simulink model "CM13_2024a_MachE_for_UA_HIL"  (R2024a)
settings: Solver=ode1  StartTime=0.0  StopTime=Inf  FixedStep=0.001  RelTol=1e-3  EnableMultiTasking=on
PreLoadFcn:
  | % if ~length(which('cmcmd')), cmenv; end
PostLoadFcn:
  | if any(exist('dsrtsu_mdlpostloadfcn', 'file') ~= 0), dsrtsu_mdlpostloadfcn('Execute', bdroot); end
InitFcn:
  | , if any(exist('rtifpga_mdlclblib', 'file') ~= 0), rtifpga_mdlclblib('Init', bdroot); end,
  | , if any(exist('dsmpb_private', 'file') ~= 0), dsmpb_private('dsmpb_mdlclblib', 'Init', bdroot); end,
values from neighbouring files (symbols this model uses):
  CoastDown =     [Run_Simulink.mat]
  limitedMCT =     [Run_Simulink.mat]
  MCT =     [Run_Simulink.mat]
  pMCT =     [Run_Simulink.mat]
  RealSimPara =     [Run_Simulink.mat]
  Ref_speed = [13 13.007895099 13.015778396 13.023649891 13.031509584 13.039357475 13.047193564 13.055017851 13.062830336 13.070631019 13.0784199 13.086196979 ... (2669 elements, 2669x1)]    [Ref_speed_and_time.mat]
  Ref_time = [0 0.01 0.02 0.03 0.04 0.05 0.06 0.07 0.08 0.09 0.1 0.11 ... (2669 elements, 2669x1)]    [Ref_speed_and_time.mat]
  US06 =     [Run_Simulink.mat]
undefined symbols (not defined in the file or in its folder): AccelCmd, ActTqLF_Nm_, ActTqLR_Nm_, ActTqRF_Nm_, ActTqRR_Nm_, BattChargeLimitMaxPwr, BattChargeLimitSocBpts, BattChargeLimitTbl, BattChrgCapcty, BattDischargeLimitSocBpts, BattDischargeLimitTbl, BattDischargeMaxPwr, BattNumCellsParallel, BattNumCellsSeries, BattOpenVoltCapBpts, BattOpenVoltTbl, BattResistSocBpts, BattResistTbl, BattResistTempBpts, BrakeMaxPrs, BrakeMaxTrq, ChassisDistCg2FrontAxle, ChassisDistCg2RearAxle, ChassisVehMass, CltchCmd, DecelCmd, DiffRatio, DiscIntNeverNeededParam, EnvGravCnst, EnvPrs, EnvTemp, FuelSpecificGrav, GearCmd, h, InitStates, lgSw, MtrEffSpdBpts, MtrEffTbl, MtrEffTrqBpts, MtrPwrMax, MtrTrqMax, planned_speed, planned_time, ref_speed, ref_time, rticanmm_blockfcn, rticanmm_initfcn, SteeringCmd, SupvsryCtrlRegenBrkCutOffTbl, SupvsryCtrlRegenSpdBpts, TestScnrioCycleNum, VEH
libraries: simulink x264, VSIGenLib x262, etargetslib x201, dsmpblib x161, CarMaker4SL x142, rtimmsu_dsrtlib x32, vehdynlibtire x24, autolibshared x19, vehdynlibsuspension x14, vehdynlibtirecommon x14, autolibutils x10, VsrLibWheel x8
(part 28 of 48)

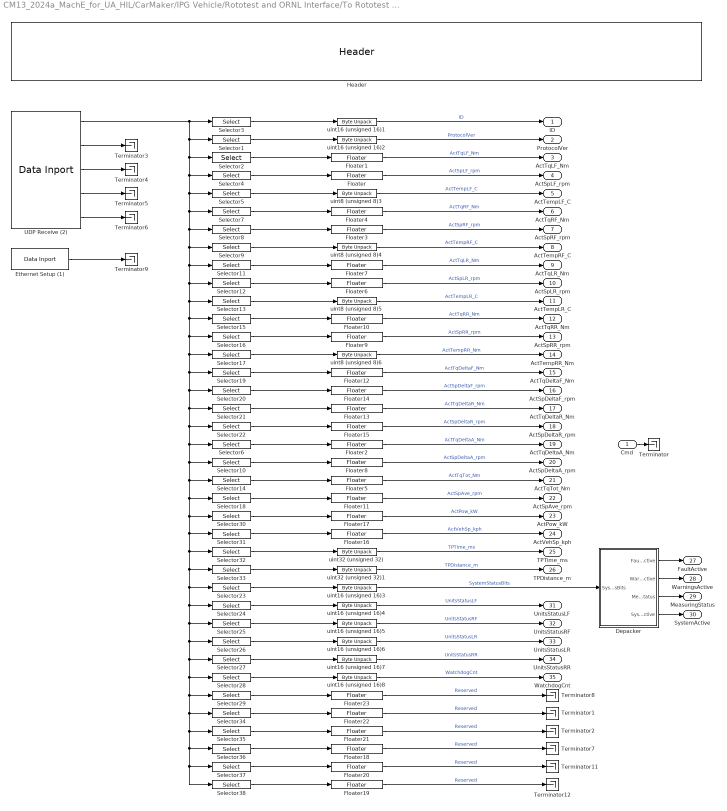
== system CM13_2024a_MachE_for_UA_HIL/CarMaker/IPG Vehicle/Rototest and ORNL Interface/To Rototest with Band-Aid/Logging/RotoTestEthRXLogging ==
  Cmd : Inport
  Depacker : Subsystem
  Ethernet Setup (1) : dsmpblib/Data Inport  Priority=10000
      settings: SourceProductName=dSPACE Model Interface Package for Simulink (MIPS)
  Floater{,1..23} (24 alike) : VSIGenLib/Floater  SystemSampleTime=-1  VariantActivationTime=update diagram  AllowFlexibleInterface=on  Latency=0  AutoFrameSizeCalculation=off
  Header : VSIGenLib/Header  not=''
  Selector1 : Selector  IndexMode=Zero-based  InputPortWidth=124  IndexOptions=Index vector (dialog)  Indices=[3 2]  OutputSizes=1
  Selector10 : Selector  IndexMode=Zero-based  InputPortWidth=124  IndexOptions=Index vector (dialog)  Indices=[63 62 61 60]  OutputSizes=1
  Selector11 : Selector  IndexMode=Zero-based  InputPortWidth=124  IndexOptions=Index vector (dialog)  Indices=[25 24 23 22]  OutputSizes=1
  Selector12 : Selector  IndexMode=Zero-based  InputPortWidth=124  IndexOptions=Index vector (dialog)  Indices=[29 28 27 26]  OutputSizes=1
  Selector13 : Selector  IndexMode=Zero-based  InputPortWidth=124  IndexOptions=Index vector (dialog)  Indices=[30]  OutputSizes=1
  Selector14 : Selector  IndexMode=Zero-based  InputPortWidth=124  IndexOptions=Index vector (dialog)  Indices=[67 66 65 64]  OutputSizes=1
  Selector15 : Selector  IndexMode=Zero-based  InputPortWidth=124  IndexOptions=Index vector (dialog)  Indices=[34 33 32 31]  OutputSizes=1
  Selector16 : Selector  IndexMode=Zero-based  InputPortWidth=124  IndexOptions=Index vector (dialog)  Indices=[38 37 36 35]  OutputSizes=1
  Selector17 : Selector  IndexMode=Zero-based  InputPortWidth=124  IndexOptions=Index vector (dialog)  Indices=[39]  OutputSizes=1
  Selector18 : Selector  IndexMode=Zero-based  InputPortWidth=124  IndexOptions=Index vector (dialog)  Indices=[71 70 69 68]  OutputSizes=1
  Selector19 : Selector  IndexMode=Zero-based  InputPortWidth=124  IndexOptions=Index vector (dialog)  Indices=[43 42 41 40]  OutputSizes=1
  Selector2 : Selector  IndexMode=Zero-based  InputPortWidth=124  IndexOptions=Index vector (dialog)  Indices=[7 6 5 4]  OutputSizes=1
  Selector20 : Selector  IndexMode=Zero-based  InputPortWidth=124  IndexOptions=Index vector (dialog)  Indices=[47 46 45 44]  OutputSizes=1
  Selector21 : Selector  IndexMode=Zero-based  InputPortWidth=124  IndexOptions=Index vector (dialog)  Indices=[51 50 49 48]  OutputSizes=1
  Selector22 : Selector  IndexMode=Zero-based  InputPortWidth=124  IndexOptions=Index vector (dialog)  Indices=[55 54 53 52]  OutputSizes=1
  Selector23 : Selector  IndexMode=Zero-based  InputPortWidth=124  IndexOptions=Index vector (dialog)  Indices=[89 88]  OutputSizes=1
  Selector24 : Selector  IndexMode=Zero-based  InputPortWidth=124  IndexOptions=Index vector (dialog)  Indices=[91 90]  OutputSizes=1
  Selector25 : Selector  IndexMode=Zero-based  InputPortWidth=124  IndexOptions=Index vector (dialog)  Indices=[93 92]  OutputSizes=1
  Selector26 : Selector  IndexMode=Zero-based  InputPortWidth=124  IndexOptions=Index vector (dialog)  Indices=[95 94]  OutputSizes=1
  Selector27 : Selector  IndexMode=Zero-based  InputPortWidth=124  IndexOptions=Index vector (dialog)  Indices=[97 96]  OutputSizes=1
  Selector28 : Selector  IndexMode=Zero-based  InputPortWidth=124  IndexOptions=Index vector (dialog)  Indices=[99 98]  OutputSizes=1
  Selector29 : Selector  IndexMode=Zero-based  InputPortWidth=124  IndexOptions=Index vector (dialog)  Indices=[103 102 101 100]  OutputSizes=1
  Selector3 : Selector  IndexMode=Zero-based  InputPortWidth=124  IndexOptions=Index vector (dialog)  Indices=[1 0]  OutputSizes=1
  Selector30 : Selector  IndexMode=Zero-based  InputPortWidth=124  IndexOptions=Index vector (dialog)  Indices=[67 66 65 64]  OutputSizes=1
  Selector31 : Selector  IndexMode=Zero-based  InputPortWidth=124  IndexOptions=Index vector (dialog)  Indices=[71 70 69 68]  OutputSizes=1
  Selector32 : Selector  IndexMode=Zero-based  InputPortWidth=124  IndexOptions=Index vector (dialog)  Indices=[83 82 81 80]  OutputSizes=1
  Selector33 : Selector  IndexMode=Zero-based  InputPortWidth=124  IndexOptions=Index vector (dialog)  Indices=[87 86 85 84]  OutputSizes=1
  Selector34 : Selector  IndexMode=Zero-based  InputPortWidth=124  IndexOptions=Index vector (dialog)  Indices=[107 106 105 104]  OutputSizes=1
  Selector35 : Selector  IndexMode=Zero-based  InputPortWidth=124  IndexOptions=Index vector (dialog)  Indices=[111 110 109 108]  OutputSizes=1
  Selector36 : Selector  IndexMode=Zero-based  InputPortWidth=124  IndexOptions=Index vector (dialog)  Indices=[115 114 113 112]  OutputSizes=1
  Selector37 : Selector  IndexMode=Zero-based  InputPortWidth=124  IndexOptions=Index vector (dialog)  Indices=[119 118 117 116]  OutputSizes=1
  Selector38 : Selector  IndexMode=Zero-based  InputPortWidth=124  IndexOptions=Index vector (dialog)  Indices=[123 122 121 120]  OutputSizes=1
  Selector4 : Selector  IndexMode=Zero-based  InputPortWidth=124  IndexOptions=Index vector (dialog)  Indices=[11 10 9 8]  OutputSizes=1
  Selector5 : Selector  IndexMode=Zero-based  InputPortWidth=124  IndexOptions=Index vector (dialog)  Indices=[12]  OutputSizes=1
  Selector6 : Selector  IndexMode=Zero-based  InputPortWidth=124  IndexOptions=Index vector (dialog)  Indices=[59 58 57 56]  OutputSizes=1
  Selector7 : Selector  IndexMode=Zero-based  InputPortWidth=124  IndexOptions=Index vector (dialog)  Indices=[16 15 14 13]  OutputSizes=1
  Selector8 : Selector  IndexMode=Zero-based  InputPortWidth=124  IndexOptions=Index vector (dialog)  Indices=[20 19 18 17]  OutputSizes=1
  Selector9 : Selector  IndexMode=Zero-based  InputPortWidth=124  IndexOptions=Index vector (dialog)  Indices=[21]  OutputSizes=1
  Terminator{,1..9,11..12} (12 alike) : Terminator
  UDP Receive (2) : dsmpblib/Data Inport  Priority=10000
      settings: SourceProductName=dSPACE Model Interface Package for Simulink (MIPS)
  uint16 (unsigned 16){1..8} (8 alike) : etargetslib/Byte Unpack  dimensions={[1]}  datatypes={'uint16'}  byteAlign=1
  uint32 (unsigned 32) : etargetslib/Byte Unpack  dimensions={[1]}  datatypes={'uint32'}  byteAlign=1
  uint32 (unsigned 32)1 : etargetslib/Byte Unpack  dimensions={[1]}  datatypes={'uint32'}  byteAlign=1
  uint8 (unsigned 8){3..6} (4 alike) : etargetslib/Byte Unpack  dimensions={[1]}  datatypes={'uint8'}  byteAlign=1
  ID : Outport
  ProtocolVer : Outport  Port=2
  ActTqLF_Nm : Outport  Port=3
  ActSpLF_rpm : Outport  Port=4
  ActTempLF_C : Outport  Port=5
  ActTqRF_Nm : Outport  Port=6
  ActSpRF_rpm : Outport  Port=7
  ActTempRF_C : Outport  Port=8
  ActTqLR_Nm : Outport  Port=9
  ActSpLR_rpm : Outport  Port=10
  ActTempLR_C : Outport  Port=11
  ActTqRR_Nm : Outport  Port=12
  ActSpRR_rpm : Outport  Port=13
  ActTempRR_Nm : Outport  Port=14
  ActTqDeltaF_Nm : Outport  Port=15
  ActSpDeltaF_rpm : Outport  Port=16
  ActTqDeltaR_Nm : Outport  Port=17
  ActSpDeltaR_rpm : Outport  Port=18
  ActTqDeltaA_Nm : Outport  Port=19
  ActSpDeltaA_rpm : Outport  Port=20
  ActTqTot_Nm : Outport  Port=21
  ActSpAve_rpm : Outport  Port=22
  ActPow_kW : Outport  Port=23
  ActVehSp_kph : Outport  Port=24
  TPTime_ms : Outport  Port=25
  TPDistance_m : Outport  Port=26
  FaultActive : Outport  Port=27
  WarningsActive : Outport  Port=28
  MeasuringStatus : Outport  Port=29
  SystemActive : Outport  Port=30
  UnitsStatusLF : Outport  Port=31
  UnitsStatusRF : Outport  Port=32
  UnitsStatusLR : Outport  Port=33
  UnitsStatusRR : Outport  Port=34
  WatchdogCnt : Outport  Port=35
  wires:
  Selector11/1 -> Floater7/1
  Floater10/1 -> ActTqRR_Nm/1  "ActTqRR_Nm"
  Selector4/1 -> Floater/1
  UDP Receive (2)/5 -> Terminator6/1
  Selector1/1 -> uint16 (unsigned 16)2/1
  Selector19/1 -> Floater12/1
  Selector21/1 -> Floater13/1
  Selector28/1 -> uint16 (unsigned 16)8/1
  UDP Receive (2)/4 -> Terminator5/1
  Selector3/1 -> uint16 (unsigned 16)1/1
  uint8 (unsigned 8)5/1 -> ActTempLR_C/1  "ActTempLR_C"
  Selector16/1 -> Floater9/1
  Selector15/1 -> Floater10/1
  Selector5/1 -> uint8 (unsigned 8)3/1
  Selector9/1 -> uint8 (unsigned 8)4/1
  Selector20/1 -> Floater14/1
  Floater6/1 -> ActSpLR_rpm/1  "ActSpLR_rpm"
  uint8 (unsigned 8)6/1 -> ActTempRR_Nm/1  "ActTempRR_Nm"
  Selector29/1 -> Floater23/1
  Floater4/1 -> ActTqRF_Nm/1  "ActTqRF_Nm"
  Selector25/1 -> uint16 (unsigned 16)5/1
  UDP Receive (2)/2 -> Terminator3/1
  Floater3/1 -> ActSpRF_rpm/1  "ActSpRF_rpm"
  uint16 (unsigned 16)3/1 -> Depacker/1(SysStsBits)  "SystemStatusBits"
  Selector26/1 -> uint16 (unsigned 16)6/1
  Selector13/1 -> uint8 (unsigned 8)5/1
  Selector2/1 -> Floater1/1
  Floater13/1 -> ActTqDeltaR_Nm/1  "ActTqDeltaR_Nm"
  Selector27/1 -> uint16 (unsigned 16)7/1
  uint16 (unsigned 16)4/1 -> UnitsStatusLF/1  "UnitsStatusLF"
  UDP Receive (2)/3 -> Terminator4/1
  Selector17/1 -> uint8 (unsigned 8)6/1
  uint16 (unsigned 16)6/1 -> UnitsStatusLR/1  "UnitsStatusLR"
  Selector23/1 -> uint16 (unsigned 16)3/1
  Selector12/1 -> Floater6/1
  Selector22/1 -> Floater15/1
  uint16 (unsigned 16)7/1 -> UnitsStatusRR/1  "UnitsStatusRR"
  Selector8/1 -> Floater3/1
  Selector7/1 -> Floater4/1
  Selector24/1 -> uint16 (unsigned 16)4/1
  uint16 (unsigned 16)2/1 -> ProtocolVer/1  "ProtocolVer"
  Floater7/1 -> ActTqLR_Nm/1  "ActTqLR_Nm"
  Floater12/1 -> ActTqDeltaF_Nm/1  "ActTqDeltaF_Nm"
  uint8 (unsigned 8)3/1 -> ActTempLF_C/1  "ActTempLF_C"
  Floater1/1 -> ActTqLF_Nm/1  "ActTqLF_Nm"
  Floater9/1 -> ActSpRR_rpm/1  "ActSpRR_rpm"
  uint16 (unsigned 16)5/1 -> UnitsStatusRF/1  "UnitsStatusRF"
  Floater14/1 -> ActSpDeltaF_rpm/1  "ActSpDeltaF_rpm"
  uint16 (unsigned 16)8/1 -> WatchdogCnt/1  "WatchdogCnt"
  Floater15/1 -> ActSpDeltaR_rpm/1  "ActSpDeltaR_rpm"
  uint16 (unsigned 16)1/1 -> ID/1  "ID"
  Floater/1 -> ActSpLF_rpm/1  "ActSpLF_rpm"
  uint8 (unsigned 8)4/1 -> ActTempRF_C/1  "ActTempRF_C"
  Depacker/3(MeasuringStatus) -> MeasuringStatus/1
  Depacker/2(WarningsActive) -> WarningsActive/1
  Depacker/1(FaultActive) -> FaultActive/1
  Depacker/4(SystemActive) -> SystemActive/1
  Ethernet Setup (1)/1 -> Terminator9/1
  Floater11/1 -> ActSpAve_rpm/1  "ActSpAve_rpm"
  Floater8/1 -> ActSpDeltaA_rpm/1  "ActSpDeltaA_rpm"
  Floater2/1 -> ActTqDeltaA_Nm/1  "ActTqDeltaA_Nm"
  Selector18/1 -> Floater11/1
  Floater5/1 -> ActTqTot_Nm/1  "ActTqTot_Nm"
  Selector10/1 -> Floater8/1
  Selector14/1 -> Floater5/1
  Selector6/1 -> Floater2/1
  Selector30/1 -> Floater17/1
  Floater17/1 -> ActPow_kW/1  "ActPow_kW"
  Selector31/1 -> Floater16/1
  Floater16/1 -> ActVehSp_kph/1  "ActVehSp_kph"
  uint32 (unsigned 32)/1 -> TPTime_ms/1  "TPTime_ms"
  uint32 (unsigned 32)1/1 -> TPDistance_m/1  "TPDistance_m"
  Selector33/1 -> uint32 (unsigned 32)1/1
  Selector32/1 -> uint32 (unsigned 32)/1
  Selector34/1 -> Floater22/1
  Selector35/1 -> Floater21/1
  Selector36/1 -> Floater18/1
  Selector37/1 -> Floater20/1
  UDP Receive (2)/1 -> Selector3/1, Selector1/1, Selector2/1, Selector4/1, Selector5/1, Selector24/1, Selector28/1, Selector38/1, Selector37/1, Selector36/1, Selector35/1, Selector34/1, Selector29/1, Selector27/1, Selector26/1, Selector25/1, Selector23/1, Selector33/1, Selector32/1, Selector31/1, Selector30/1, Selector18/1, Selector14/1, Selector10/1, Selector6/1, Selector22/1, Selector21/1, Selector20/1, Selector19/1, Selector17/1, Selector16/1, Selector15/1, Selector13/1, Selector12/1, Selector11/1, Selector9/1, Selector8/1, Selector7/1
  Selector38/1 -> Floater19/1
  Floater18/1 -> Terminator7/1  "Reserved"
  Floater19/1 -> Terminator12/1  "Reserved"
  Floater20/1 -> Terminator11/1  "Reserved"
  Floater21/1 -> Terminator2/1  "Reserved"
  Floater22/1 -> Terminator1/1  "Reserved"
  Floater23/1 -> Terminator8/1  "Reserved"
  Cmd/1 -> Terminator/1

== system CM13_2024a_MachE_for_UA_HIL/CarMaker/IPG Vehicle/Rototest and ORNL Interface/To Rototest with Band-Aid/RotoTestEthTx/Packer ==
  SpTqRR : Inport
  SpTqLR : Inport  Port=2
  SpTqRF : Inport  Port=3
  SpTqLF : Inport  Port=4
  SystemActive : Inport  Port=5
  Add : Sum  Inputs=++++++++  OutDataTypeStr=uint8
  Bit0 : Gain  OutDataTypeStr=uint8
  Bit1 : Gain  Gain=2  OutDataTypeStr=uint8
  Bit2 : Gain  Gain=4  OutDataTypeStr=Inherit: Inherit via back propagation
  Bit3 : Gain  Gain=8  OutDataTypeStr=uint8
  Bit4 : Gain  Gain=16  OutDataTypeStr=uint8
  Bit5 : Gain  Gain=32  OutDataTypeStr=uint8
  Bit6 : Gain  Gain=64  OutDataTypeStr=uint8
  Bit7 : Gain  Gain=128  OutDataTypeStr=uint8
  Ground11 : Ground
  Header : VSIGenLib/Header  not=''
  SystemCtrlBits : Outport
  wires:
  Bit2/1 -> Add/6  "SpTqRF"
  Bit5/1 -> Add/3  "Reserved"
  Ground11/1 -> Bit6/1, Bit5/1, Bit7/1  "Reserved"
  Bit3/1 -> Add/5  "SpTqLR"
  Bit6/1 -> Add/2  "Reserved"
  Bit4/1 -> Add/4  "SpTqRR"
  SystemActive/1 -> Bit0/1
  Bit7/1 -> Add/1  "Reserved"
  Bit1/1 -> Add/7  "SpTqLF"
  Bit0/1 -> Add/8  "SystemActive"
  Add/1 -> SystemCtrlBits/1  "SystemCtrlBits"
  SpTqLR/1 -> Bit3/1
  SpTqRR/1 -> Bit4/1
  SpTqLF/1 -> Bit1/1
  SpTqRF/1 -> Bit2/1

== system CM13_2024a_MachE_for_UA_HIL/CarMaker/IPG Vehicle/Rototest and ORNL Interface/To Rototest with Band-Aid/SteeringSystem/RotoTestEthRX ==
  Depacker : Subsystem
  Floater{,1..2,4} (4 alike) : VSIGenLib/Floater  SystemSampleTime=-1  VariantActivationTime=update diagram  AllowFlexibleInterface=on  Latency=0  AutoFrameSizeCalculation=off
  NS System UDP Rx : dsmpblib/Data Inport  Priority=10000
      settings: SourceProductName=dSPACE Model Interface Package for Simulink (MIPS)
  NS System UDP Rx1 : dsmpblib/Data Inport  Priority=10000
      settings: SourceProductName=dSPACE Model Interface Package for Simulink (MIPS)
  Selector1 : Selector  IndexMode=Zero-based  InputPortWidth=32  IndexOptions=Index vector (dialog)  Indices=[3 2]  OutputSizes=1
  Selector2 : Selector  IndexMode=Zero-based  InputPortWidth=32  IndexOptions=Index vector (dialog)  Indices=[7 6 5 4]  OutputSizes=1
  Selector23 : Selector  IndexMode=Zero-based  InputPortWidth=32  IndexOptions=Index vector (dialog)  Indices=[25 24]  OutputSizes=1
  Selector24 : Selector  IndexMode=Zero-based  InputPortWidth=32  IndexOptions=Index vector (dialog)  Indices=[27 26]  OutputSizes=1
  Selector25 : Selector  IndexMode=Zero-based  InputPortWidth=32  IndexOptions=Index vector (dialog)  Indices=[29 28]  OutputSizes=1
  Selector28 : Selector  IndexMode=Zero-based  InputPortWidth=32  IndexOptions=Index vector (dialog)  Indices=[30]  OutputSizes=1
  Selector29 : Selector  IndexMode=Zero-based  InputPortWidth=32  IndexOptions=Index vector (dialog)  Indices=[31]  OutputSizes=1
  Selector3 : Selector  IndexMode=Zero-based  InputPortWidth=32  IndexOptions=Index vector (dialog)  Indices=[1 0]  OutputSizes=1
  Selector4 : Selector  IndexMode=Zero-based  InputPortWidth=32  IndexOptions=Index vector (dialog)  Indices=[11 10 9 8]  OutputSizes=1
  Selector5 : Selector  IndexMode=Zero-based  InputPortWidth=32  IndexOptions=Index vector (dialog)  Indices=[15 14 13 12]  OutputSizes=1
  Selector6 : Selector  IndexMode=Zero-based  InputPortWidth=32  IndexOptions=Index vector (dialog)  Indices=[19 18 17 16]  OutputSizes=1
  Selector7 : Selector  IndexMode=Zero-based  InputPortWidth=32  IndexOptions=Index vector (dialog)  Indices=[23 22 21 20]  OutputSizes=1
  Terminator{1..6,8..9} (8 alike) : Terminator
  uint16 (unsigned 16){1..5} (5 alike) : etargetslib/Byte Unpack  dimensions={[1]}  datatypes={'uint16'}  byteAlign=1
  uint32 (unsigned 32)5 : etargetslib/Byte Unpack  dimensions={[1]}  datatypes={'uint32'}  byteAlign=1
  uint8 (unsigned 8)1 : etargetslib/Byte Unpack  dimensions={[1]}  datatypes={'uint8'}  byteAlign=1
  uint8 (unsigned 8)2 : etargetslib/Byte Unpack  dimensions={[1]}  datatypes={'uint8'}  byteAlign=1
  ID : Outport
  ProtocolVer : Outport  Port=2
  ActSteerAng : Outport  Port=3
  ActAngularSp : Outport  Port=4
  RefSteerAng : Outport  Port=5
  RefAngularSp : Outport  Port=6
  WatchdogCnt : Outport  Port=7
  FaultActive : Outport  Port=8
  WarningsActive : Outport  Port=9
  InSimulationMode : Outport  Port=10
  HardLimitActive : Outport  Port=11
  SoftLimitActive : Outport  Port=12
  TeachInDone : Outport  Port=13
  Ready : Outport  Port=14
  SystemActive : Outport  Port=15
  wires:
  Depacker/8(SystemActive) -> SystemActive/1
  Depacker/6(TeachInDone) -> TeachInDone/1
  Depacker/1(FaultActive) -> FaultActive/1
  Depacker/2(WarningsActive) -> WarningsActive/1
  Depacker/7(Ready) -> Ready/1
  Floater/1 -> ActAngularSp/1  "ActAngularSp"
  Floater2/1 -> RefSteerAng/1  "RefSteerAng"
  uint16 (unsigned 16)1/1 -> ID/1  "ID"
  uint8 (unsigned 8)1/1 -> WatchdogCnt/1  "WatchdogCnt"
  uint16 (unsigned 16)5/1 -> Terminator2/1  "Reserved"
  Floater1/1 -> ActSteerAng/1  "ActSteerAng"
  uint32 (unsigned 32)5/1 -> Terminator9/1  "Reserved"
  uint16 (unsigned 16)2/1 -> ProtocolVer/1  "ProtocolVer"
  Selector24/1 -> uint16 (unsigned 16)4/1
  Selector7/1 -> Floater4/1
  Selector23/1 -> uint16 (unsigned 16)3/1
  NS System UDP Rx/3 -> Terminator4/1
  uint16 (unsigned 16)4/1 -> Terminator1/1  "Reserved"
  Selector2/1 -> Floater1/1
  Selector6/1 -> Floater2/1
  uint16 (unsigned 16)3/1 -> Depacker/1(SysStsBits)  "SystemStatusBits"
  NS System UDP Rx/2 -> Terminator3/1
  Selector25/1 -> uint16 (unsigned 16)5/1
  Floater4/1 -> RefAngularSp/1  "RefAngularSp"
  uint8 (unsigned 8)2/1 -> Terminator8/1  "Reserved"
  Selector5/1 -> uint32 (unsigned 32)5/1
  Selector3/1 -> uint16 (unsigned 16)1/1
  NS System UDP Rx/4 -> Terminator5/1
  Selector28/1 -> uint8 (unsigned 8)1/1
  Selector29/1 -> uint8 (unsigned 8)2/1
  NS System UDP Rx/1 -> Selector23/1, Selector24/1, Selector25/1, Selector29/1, Selector28/1, Selector7/1, Selector6/1, Selector5/1, Selector4/1, Selector2/1, Selector1/1, Selector3/1
  Selector1/1 -> uint16 (unsigned 16)2/1
  NS System UDP Rx/5 -> Terminator6/1
  Selector4/1 -> Floater/1
  Depacker/3(InSimulationMode) -> InSimulationMode/1
  Depacker/4(HardLimitActive) -> HardLimitActive/1
  Depacker/5(SoftLimitActive) -> SoftLimitActive/1

== system CM13_2024a_MachE_for_UA_HIL/CarMaker_new/IPG Vehicle/Actuation and Outputs/MOOG Brake Actuator/ CAN Settings/ CAN diagnostic Counter ==
  RX Counter : Inport
  Compare To Constant3 : simulink/Logic and Bit Operations/Compare To Constant  relop=<=  const=TimeOutDuration  OutDataTypeStr=boolean
  Memory2 : Memory  InheritSampleTime=on
  Relational Operator2 : RelationalOperator  Operator=~=  OutDataTypeStr=boolean  InputSameDT=off
  Timer : Subsystem
  CommsOKFlag : Outport
  wires:
  Relational Operator2/1 -> Timer/1(Reset)
  Timer/1(Timer) -> Compare To Constant3/1
  RX Counter/1 -> Relational Operator2/1, Memory2/1
  Memory2/1 -> Relational Operator2/2
  Compare To Constant3/1 -> CommsOKFlag/1

== system CM13_2024a_MachE_for_UA_HIL/CarMaker_new/IPG Vehicle/Actuation and Outputs/MOOG Brake Actuator/MOOG Interface/Max Stop Adjustment ==
  In1 : Inport
  Enable : EnablePort
  MaxStopOffset : Constant  Value=-3500
  Sum3 : Sum  Inputs=|++
  Out1 : Outport  InitialOutput=[0]
  wires:
  MaxStopOffset/1 -> Sum3/2
  In1/1 -> Sum3/1
  Sum3/1 -> Out1/1

== system CM13_2024a_MachE_for_UA_HIL/CarMaker_new/IPG Vehicle/Actuation and Outputs/MOOG Brake Actuator/MOOG Interface/Min Stop Adjustment ==
  In1 : Inport
  Enable : EnablePort
  MinStopOffset : Constant  Value=4100
  Sum3 : Sum  Inputs=|++
  Out1 : Outport  InitialOutput=[0]
  wires:
  In1/1 -> Sum3/1
  Sum3/1 -> Out1/1
  MinStopOffset/1 -> Sum3/2

== system CM13_2024a_MachE_for_UA_HIL/CarMaker_new/IPG Vehicle/Actuation and Outputs/MOOG Brake Actuator/MOOG Interface/Rising edge ==
  In : Inport
  Memory : Memory  InheritSampleTime=on
  Sum3 : Sum  Inputs=|+-
  Out : Outport
  wires:
  In/1 -> Memory/1, Sum3/1
  Memory/1 -> Sum3/2
  Sum3/1 -> Out/1

== system CM13_2024a_MachE_for_UA_HIL/CarMaker_new/IPG Vehicle/Actuation and Outputs/MOOG Brake Actuator/MOOG Interface/Rising edge1 ==
  In : Inport
  Memory : Memory  InheritSampleTime=on
  Sum3 : Sum  Inputs=|+-
  Out : Outport
  wires:
  In/1 -> Memory/1, Sum3/1
  Memory/1 -> Sum3/2
  Sum3/1 -> Out/1

== system CM13_2024a_MachE_for_UA_HIL/CarMaker_new/IPG Vehicle/CarAndTrailer/Forces/Tires/TireFL ==
  note: Insert your tire model here.
  Sync_In : Inport
  Load : Inport  Port=2
  vxtrans : Inport  Port=3
  vytrans : Inport  Port=4
  Rim_rotv : Inport  Port=5
  Rim_turnv : Inport  Port=6
  InclinAngle : Inport  Port=7
  muRoad : Inport  Port=8
  Ground{1..11} (11 alike) : Ground
  Terminator{,1..6,12} (8 alike) : Terminator
  Slp : Outport  VectorParamsAs1DForOutWhenUnconnected=off
  Alpha : Outport  Port=2  VectorParamsAs1DForOutWhenUnconnected=off
  TurnSlp : Outport  Port=3  VectorParamsAs1DForOutWhenUnconnected=off
  rBelt_eff : Outport  Port=4  VectorParamsAs1DForOutWhenUnconnected=off
  vBelt : Outport  Port=5  VectorParamsAs1DForOutWhenUnconnected=off
  LongFrc : Outport  Port=6  VectorParamsAs1DForOutWhenUnconnected=off
  SideFrc : Outport  Port=7  VectorParamsAs1DForOutWhenUnconnected=off
  LoadFrc : Outport  Port=8  VectorParamsAs1DForOutWhenUnconnected=off
  OverturnTrq : Outport  Port=9  VectorParamsAs1DForOutWhenUnconnected=off
  RollResist : Outport  Port=10  VectorParamsAs1DForOutWhenUnconnected=off
  AlignTrq : Outport  Port=11  VectorParamsAs1DForOutWhenUnconnected=off
  wires:
  Ground11/1 -> vBelt/1
  Ground10/1 -> rBelt_eff/1
  Ground9/1 -> TurnSlp/1
  Rim_turnv/1 -> Terminator6/1
  Sync_In/1 -> Terminator12/1
  Ground2/1 -> Alpha/1
  Ground3/1 -> LongFrc/1
  Ground4/1 -> SideFrc/1
  Ground5/1 -> OverturnTrq/1
  vxtrans/1 -> Terminator1/1
  vytrans/1 -> Terminator2/1
  Rim_rotv/1 -> Terminator3/1
  InclinAngle/1 -> Terminator4/1
  muRoad/1 -> Terminator5/1
  Load/1 -> Terminator/1
  Ground1/1 -> Slp/1
  Ground6/1 -> LoadFrc/1
  Ground7/1 -> RollResist/1
  Ground8/1 -> AlignTrq/1

== system CM13_2024a_MachE_for_UA_HIL/CarMaker_new/IPG Vehicle/CarAndTrailer/Forces/Tires/TireFR ==
  note: Insert your tire model here.
  Sync_In : Inport
  Load : Inport  Port=2
  vxtrans : Inport  Port=3
  vytrans : Inport  Port=4
  Rim_rotv : Inport  Port=5
  Rim_turnv : Inport  Port=6
  InclinAngle : Inport  Port=7
  muRoad : Inport  Port=8
  Ground{1..11} (11 alike) : Ground
  Terminator{,1..6,12} (8 alike) : Terminator
  Slp : Outport  VectorParamsAs1DForOutWhenUnconnected=off
  Alpha : Outport  Port=2  VectorParamsAs1DForOutWhenUnconnected=off
  TurnSlp : Outport  Port=3  VectorParamsAs1DForOutWhenUnconnected=off
  rBelt_eff : Outport  Port=4  VectorParamsAs1DForOutWhenUnconnected=off
  vBelt : Outport  Port=5  VectorParamsAs1DForOutWhenUnconnected=off
  LongFrc : Outport  Port=6  VectorParamsAs1DForOutWhenUnconnected=off
  SideFrc : Outport  Port=7  VectorParamsAs1DForOutWhenUnconnected=off
  LoadFrc : Outport  Port=8  VectorParamsAs1DForOutWhenUnconnected=off
  OverturnTrq : Outport  Port=9  VectorParamsAs1DForOutWhenUnconnected=off
  RollResist : Outport  Port=10  VectorParamsAs1DForOutWhenUnconnected=off
  AlignTrq : Outport  Port=11  VectorParamsAs1DForOutWhenUnconnected=off
  wires:
  Ground11/1 -> vBelt/1
  Ground10/1 -> rBelt_eff/1
  Ground9/1 -> TurnSlp/1
  Rim_turnv/1 -> Terminator6/1
  Sync_In/1 -> Terminator12/1
  Ground2/1 -> Alpha/1
  Ground3/1 -> LongFrc/1
  Ground4/1 -> SideFrc/1
  Ground5/1 -> OverturnTrq/1
  vxtrans/1 -> Terminator1/1
  vytrans/1 -> Terminator2/1
  Rim_rotv/1 -> Terminator3/1
  InclinAngle/1 -> Terminator4/1
  muRoad/1 -> Terminator5/1
  Load/1 -> Terminator/1
  Ground1/1 -> Slp/1
  Ground6/1 -> LoadFrc/1
  Ground7/1 -> RollResist/1
  Ground8/1 -> AlignTrq/1

== system CM13_2024a_MachE_for_UA_HIL/CarMaker_new/IPG Vehicle/CarAndTrailer/Forces/Tires/TireRL ==
  note: Insert your tire model here.
  Sync_In : Inport
  Load : Inport  Port=2
  vxtrans : Inport  Port=3
  vytrans : Inport  Port=4
  Rim_rotv : Inport  Port=5
  Rim_turnv : Inport  Port=6
  InclinAngle : Inport  Port=7
  muRoad : Inport  Port=8
  Ground{1..11} (11 alike) : Ground
  Terminator{,1..6,12} (8 alike) : Terminator
  Slp : Outport  VectorParamsAs1DForOutWhenUnconnected=off
  Alpha : Outport  Port=2  VectorParamsAs1DForOutWhenUnconnected=off
  TurnSlp : Outport  Port=3  VectorParamsAs1DForOutWhenUnconnected=off
  rBelt_eff : Outport  Port=4  VectorParamsAs1DForOutWhenUnconnected=off
  vBelt : Outport  Port=5  VectorParamsAs1DForOutWhenUnconnected=off
  LongFrc : Outport  Port=6  VectorParamsAs1DForOutWhenUnconnected=off
  SideFrc : Outport  Port=7  VectorParamsAs1DForOutWhenUnconnected=off
  LoadFrc : Outport  Port=8  VectorParamsAs1DForOutWhenUnconnected=off
  OverturnTrq : Outport  Port=9  VectorParamsAs1DForOutWhenUnconnected=off
  RollResist : Outport  Port=10  VectorParamsAs1DForOutWhenUnconnected=off
  AlignTrq : Outport  Port=11  VectorParamsAs1DForOutWhenUnconnected=off
  wires:
  Ground11/1 -> vBelt/1
  Ground10/1 -> rBelt_eff/1
  Ground9/1 -> TurnSlp/1
  Rim_turnv/1 -> Terminator6/1
  Sync_In/1 -> Terminator12/1
  Ground2/1 -> Alpha/1
  Ground3/1 -> LongFrc/1
  Ground4/1 -> SideFrc/1
  Ground5/1 -> OverturnTrq/1
  vxtrans/1 -> Terminator1/1
  vytrans/1 -> Terminator2/1
  Rim_rotv/1 -> Terminator3/1
  InclinAngle/1 -> Terminator4/1
  muRoad/1 -> Terminator5/1
  Load/1 -> Terminator/1
  Ground1/1 -> Slp/1
  Ground6/1 -> LoadFrc/1
  Ground7/1 -> RollResist/1
  Ground8/1 -> AlignTrq/1

== system CM13_2024a_MachE_for_UA_HIL/CarMaker_new/IPG Vehicle/CarAndTrailer/Forces/Tires/TireRR ==
  note: Insert your tire model here.
  Sync_In : Inport
  Load : Inport  Port=2
  vxtrans : Inport  Port=3
  vytrans : Inport  Port=4
  Rim_rotv : Inport  Port=5
  Rim_turnv : Inport  Port=6
  InclinAngle : Inport  Port=7
  muRoad : Inport  Port=8
  Ground{1..11} (11 alike) : Ground
  Terminator{,1..6,12} (8 alike) : Terminator
  Slp : Outport  VectorParamsAs1DForOutWhenUnconnected=off
  Alpha : Outport  Port=2  VectorParamsAs1DForOutWhenUnconnected=off
  TurnSlp : Outport  Port=3  VectorParamsAs1DForOutWhenUnconnected=off
  rBelt_eff : Outport  Port=4  VectorParamsAs1DForOutWhenUnconnected=off
  vBelt : Outport  Port=5  VectorParamsAs1DForOutWhenUnconnected=off
  LongFrc : Outport  Port=6  VectorParamsAs1DForOutWhenUnconnected=off
  SideFrc : Outport  Port=7  VectorParamsAs1DForOutWhenUnconnected=off
  LoadFrc : Outport  Port=8  VectorParamsAs1DForOutWhenUnconnected=off
  OverturnTrq : Outport  Port=9  VectorParamsAs1DForOutWhenUnconnected=off
  RollResist : Outport  Port=10  VectorParamsAs1DForOutWhenUnconnected=off
  AlignTrq : Outport  Port=11  VectorParamsAs1DForOutWhenUnconnected=off
  wires:
  Ground11/1 -> vBelt/1
  Ground10/1 -> rBelt_eff/1
  Ground9/1 -> TurnSlp/1
  Rim_turnv/1 -> Terminator6/1
  Sync_In/1 -> Terminator12/1
  Ground2/1 -> Alpha/1
  Ground3/1 -> LongFrc/1
  Ground4/1 -> SideFrc/1
  Ground5/1 -> OverturnTrq/1
  vxtrans/1 -> Terminator1/1
  vytrans/1 -> Terminator2/1
  Rim_rotv/1 -> Terminator3/1
  InclinAngle/1 -> Terminator4/1
  muRoad/1 -> Terminator5/1
  Load/1 -> Terminator/1
  Ground1/1 -> Slp/1
  Ground6/1 -> LoadFrc/1
  Ground7/1 -> RollResist/1
  Ground8/1 -> AlignTrq/1

== system CM13_2024a_MachE_for_UA_HIL/CarMaker_new/IPG Vehicle/Mach-E CAN BM/Subsystem/Logic/UnitConversion ==
  In1 : Inport
  Bus Creator : BusCreator  Inputs=5
  busselector2 : BusSelector  OutputSignals=RollRate_Vehicle_CoG[rad|s],YawRate_Vehicle_CoG[rad|s],a_x_Vehicle_CoG_withG[m|s2],a_y_Vehicle_CoG_withG[m|s2],a_z_Vehicle_CoG_withG[m|s2]
  deg to rad{,1..3} (4 alike) : Gain
  deg to rad_ : Gain
  Out1 : Outport  VectorParamsAs1DForOutWhenUnconnected=off
  wires:
  deg to rad3/1 -> Bus Creator/5  "a_z_Vehicle_CoG_withG[m|s2]"
  deg to rad2/1 -> Bus Creator/4  "a_y_Vehicle_CoG_withG[m|s2]"
  deg to rad1/1 -> Bus Creator/3  "a_x_Vehicle_CoG_withG[m|s2]"
  busselector2/5 -> deg to rad3/1  "<a_z_Vehicle_CoG_withG[m|s2]>"
  busselector2/4 -> deg to rad2/1  "<a_y_Vehicle_CoG_withG[m|s2]>"
  busselector2/3 -> deg to rad1/1  "<a_x_Vehicle_CoG_withG[m|s2]>"
  Bus Creator/1 -> Out1/1  "UnitConversion"
  deg to rad/1 -> Bus Creator/2  "YawRate_Vehicle_CoG[rad|s]"
  deg to rad_/1 -> Bus Creator/1  "RollRate_Vehicle_CoG[rad|s]"
  In1/1 -> busselector2/1
  busselector2/1 -> deg to rad_/1  "<RollRate_Vehicle_CoG[rad|s]>"
  busselector2/2 -> deg to rad/1  "<YawRate_Vehicle_CoG[rad|s]>"

== system CM13_2024a_MachE_for_UA_HIL/CarMaker_new/IPG Vehicle/Mach-E CAN BM/Subsystem1/Logic/UnitConversion ==
  In1 : Inport
  Bus Creator : BusCreator  Inputs=5
  busselector2 : BusSelector  OutputSignals=RollRate_Vehicle_CoG[rad|s],YawRate_Vehicle_CoG[rad|s],a_x_Vehicle_CoG_withG[m|s2],a_y_Vehicle_CoG_withG[m|s2],a_z_Vehicle_CoG_withG[m|s2]
  deg to rad{,1..3} (4 alike) : Gain
  deg to rad_ : Gain
  Out1 : Outport  VectorParamsAs1DForOutWhenUnconnected=off
  wires:
  deg to rad3/1 -> Bus Creator/5  "a_z_Vehicle_CoG_withG[m|s2]"
  deg to rad2/1 -> Bus Creator/4  "a_y_Vehicle_CoG_withG[m|s2]"
  deg to rad1/1 -> Bus Creator/3  "a_x_Vehicle_CoG_withG[m|s2]"
  busselector2/5 -> deg to rad3/1  "<a_z_Vehicle_CoG_withG[m|s2]>"
  busselector2/4 -> deg to rad2/1  "<a_y_Vehicle_CoG_withG[m|s2]>"
  busselector2/3 -> deg to rad1/1  "<a_x_Vehicle_CoG_withG[m|s2]>"
  Bus Creator/1 -> Out1/1  "UnitConversion"
  deg to rad/1 -> Bus Creator/2  "YawRate_Vehicle_CoG[rad|s]"
  deg to rad_/1 -> Bus Creator/1  "RollRate_Vehicle_CoG[rad|s]"
  In1/1 -> busselector2/1
  busselector2/1 -> deg to rad_/1  "<RollRate_Vehicle_CoG[rad|s]>"
  busselector2/2 -> deg to rad/1  "<YawRate_Vehicle_CoG[rad|s]>"

== system CM13_2024a_MachE_for_UA_HIL/CarMaker_new/IPG Vehicle/MachE CAN/Subsystem/Logic/UnitConversion ==
  In1 : Inport
  Bus Creator : BusCreator  Inputs=5
  busselector2 : BusSelector  OutputSignals=RollRate_Vehicle_CoG[rad|s],YawRate_Vehicle_CoG[rad|s],a_x_Vehicle_CoG_withG[m|s2],a_y_Vehicle_CoG_withG[m|s2],a_z_Vehicle_CoG_withG[m|s2]
  deg to rad{,1..3} (4 alike) : Gain
  deg to rad_ : Gain
  Out1 : Outport  VectorParamsAs1DForOutWhenUnconnected=off
  wires:
  deg to rad3/1 -> Bus Creator/5  "a_z_Vehicle_CoG_withG[m|s2]"
  deg to rad2/1 -> Bus Creator/4  "a_y_Vehicle_CoG_withG[m|s2]"
  deg to rad1/1 -> Bus Creator/3  "a_x_Vehicle_CoG_withG[m|s2]"
  busselector2/5 -> deg to rad3/1  "<a_z_Vehicle_CoG_withG[m|s2]>"
  busselector2/4 -> deg to rad2/1  "<a_y_Vehicle_CoG_withG[m|s2]>"
  busselector2/3 -> deg to rad1/1  "<a_x_Vehicle_CoG_withG[m|s2]>"
  Bus Creator/1 -> Out1/1  "UnitConversion"
  deg to rad/1 -> Bus Creator/2  "YawRate_Vehicle_CoG[rad|s]"
  deg to rad_/1 -> Bus Creator/1  "RollRate_Vehicle_CoG[rad|s]"
  In1/1 -> busselector2/1
  busselector2/1 -> deg to rad_/1  "<RollRate_Vehicle_CoG[rad|s]>"
  busselector2/2 -> deg to rad/1  "<YawRate_Vehicle_CoG[rad|s]>"

== system CM13_2024a_MachE_for_UA_HIL/CarMaker_new/IPG Vehicle/MachE CAN/Subsystem/Mapping/Accel_Data ==
  In1 : Inport
  Gain : Gain
  Gain1 : Gain
  Gain2 : Gain
  buscreator : BusCreator  Inputs=3
  busselector : BusSelector  OutputSignals=a_y_Vehicle_CoG_withG[m|s2],a_x_Vehicle_CoG_withG[m|s2],a_z_Vehicle_CoG_withG[m|s2]
  Out1 : Outport  VectorParamsAs1DForOutWhenUnconnected=off
  wires:
  Gain2/1 -> buscreator/3  "VehVert2_A_Actl"
  Gain1/1 -> buscreator/2  "VehLong2_A_Actl"
  Gain/1 -> buscreator/1  "VehLat2_A_Actl"
  busselector/1 -> Gain/1  "<a_y_Vehicle_CoG_withG[m|s2]>"
  busselector/2 -> Gain1/1  "<a_x_Vehicle_CoG_withG[m|s2]>"
  busselector/3 -> Gain2/1  "<a_z_Vehicle_CoG_withG[m|s2]>"
  buscreator/1 -> Out1/1  "Accel_Data"
  In1/1 -> busselector/1

== system CM13_2024a_MachE_for_UA_HIL/CarMaker_new/IPG Vehicle/MachE CAN/Subsystem/Mapping/Yaw_Data ==
  In1 : Inport
  Gain : Gain
  Gain1 : Gain
  buscreator : BusCreator  Inputs=2
  busselector : BusSelector  OutputSignals=RollRate_Vehicle_CoG[rad|s],YawRate_Vehicle_CoG[rad|s]
  Out1 : Outport  VectorParamsAs1DForOutWhenUnconnected=off
  wires:
  busselector/1 -> Gain/1  "<RollRate_Vehicle_CoG[rad|s]>"
  busselector/2 -> Gain1/1  "<YawRate_Vehicle_CoG[rad|s]>"
  Gain1/1 -> buscreator/2  "VehYaw_W_Actl"
  In1/1 -> busselector/1
  buscreator/1 -> Out1/1  "Yaw_Data"
  Gain/1 -> buscreator/1  "VehRol_W_Actl"

== system CM13_2024a_MachE_for_UA_HIL/CarMaker_new/IPG Vehicle/Rototest and ORNL Interface/From Rototest/RotoTestEthRX/Depacker ==
  SysStsBits : Inport
  Extract Bits1 : simulink/Logic and Bit Operations/Extract Bits  bitsToExtract=Range of bits  numBits=8  bitIdxRange=[7]  outScalingMode=Preserve fixed-point scaling
  Extract Bits10 : simulink/Logic and Bit Operations/Extract Bits  bitsToExtract=Range of bits  numBits=8  bitIdxRange=[9]  outScalingMode=Preserve fixed-point scaling
  Extract Bits11 : simulink/Logic and Bit Operations/Extract Bits  bitsToExtract=Range of bits  numBits=8  bitIdxRange=[10]  outScalingMode=Preserve fixed-point scaling
  Extract Bits12 : simulink/Logic and Bit Operations/Extract Bits  bitsToExtract=Range of bits  numBits=8  bitIdxRange=[11]  outScalingMode=Preserve fixed-point scaling
  Extract Bits13 : simulink/Logic and Bit Operations/Extract Bits  bitsToExtract=Range of bits  numBits=8  bitIdxRange=[12]  outScalingMode=Preserve fixed-point scaling
  Extract Bits14 : simulink/Logic and Bit Operations/Extract Bits  bitsToExtract=Range of bits  numBits=8  bitIdxRange=[13]  outScalingMode=Preserve fixed-point scaling
  Extract Bits15 : simulink/Logic and Bit Operations/Extract Bits  bitsToExtract=Range of bits  numBits=8  bitIdxRange=[14]  outScalingMode=Preserve fixed-point scaling
  Extract Bits16 : simulink/Logic and Bit Operations/Extract Bits  bitsToExtract=Range of bits  numBits=8  bitIdxRange=[15]  outScalingMode=Preserve fixed-point scaling
  Extract Bits2 : simulink/Logic and Bit Operations/Extract Bits  bitsToExtract=Range of bits  numBits=8  bitIdxRange=[6]  outScalingMode=Preserve fixed-point scaling
  Extract Bits3 : simulink/Logic and Bit Operations/Extract Bits  bitsToExtract=Range of bits  numBits=8  bitIdxRange=[5]  outScalingMode=Preserve fixed-point scaling
  Extract Bits4 : simulink/Logic and Bit Operations/Extract Bits  bitsToExtract=Range of bits  numBits=8  bitIdxRange=[4]  outScalingMode=Preserve fixed-point scaling
  Extract Bits5 : simulink/Logic and Bit Operations/Extract Bits  bitsToExtract=Range of bits  numBits=8  bitIdxRange=[3]  outScalingMode=Preserve fixed-point scaling
  Extract Bits6 : simulink/Logic and Bit Operations/Extract Bits  bitsToExtract=Range of bits  numBits=8  bitIdxRange=[2]  outScalingMode=Preserve fixed-point scaling
  Extract Bits7 : simulink/Logic and Bit Operations/Extract Bits  bitsToExtract=Range of bits  numBits=8  bitIdxRange=[1]  outScalingMode=Preserve fixed-point scaling
  Extract Bits8 : simulink/Logic and Bit Operations/Extract Bits  bitsToExtract=Range of bits  numBits=8  bitIdxRange=[0]  outScalingMode=Preserve fixed-point scaling
  Extract Bits9 : simulink/Logic and Bit Operations/Extract Bits  bitsToExtract=Range of bits  numBits=8  bitIdxRange=[8]  outScalingMode=Preserve fixed-point scaling
  Gain : Gain  Gain=1/128
  Gain1 : Gain  Gain=1/64
  Gain10 : Gain  Gain=1/1024
  Gain11 : Gain  Gain=1/2048
  Gain12 : Gain  Gain=1/4096
  Gain13 : Gain  Gain=1/8192
  Gain14 : Gain  Gain=1/16384
  Gain15 : Gain  Gain=1/32768
  Gain2 : Gain  Gain=1/32
  Gain3 : Gain  Gain=1/16
  Gain4 : Gain  Gain=1/8
  Gain5 : Gain  Gain=1/4
  Gain6 : Gain  Gain=1/2
  Gain7 : Gain  Gain=1/1
  Gain8 : Gain  Gain=1/256
  Gain9 : Gain  Gain=1/512
  Header : VSIGenLib/Header  not=''
  Terminator{,1..8} (9 alike) : Terminator
  FaultActive : Outport
  WarningsActive : Outport  Port=2
  SpTqRR : Outport  Port=3
  SpTqLR : Outport  Port=4
  SpTqRF : Outport  Port=5
  SpTqLF : Outport  Port=6
  SystemActive : Outport  Port=7
  wires:
  Gain5/1 -> Terminator3/1  "Reserved"
  Gain6/1 -> Terminator4/1  "Reserved"
  Gain3/1 -> Terminator1/1  "Reserved"
  Gain4/1 -> Terminator2/1  "Reserved"
  Gain2/1 -> Terminator/1  "Reserved"
  Gain1/1 -> WarningsActive/1  "WarningsActive"
  Gain/1 -> FaultActive/1  "FaultActive"
  Gain7/1 -> Terminator5/1  "Reserved"
  Gain8/1 -> SystemActive/1  "SystemActive"
  Gain9/1 -> SpTqLF/1  "SpTqLF"
  Gain10/1 -> SpTqRF/1  "SpTqRF"
  Gain11/1 -> SpTqLR/1  "SpTqLR"
  Gain12/1 -> SpTqRR/1  "SpTqRR"
  Gain14/1 -> Terminator7/1  "Reserved"
  Gain13/1 -> Terminator8/1  "Reserved"
  Gain15/1 -> Terminator6/1  "Reserved"
  SysStsBits/1 -> Extract Bits9/1, Extract Bits10/1, Extract Bits16/1, Extract Bits15/1, Extract Bits14/1, Extract Bits13/1, Extract Bits12/1, Extract Bits11/1, Extract Bits8/1, Extract Bits7/1, Extract Bits6/1, Extract Bits5/1, Extract Bits4/1, Extract Bits3/1, Extract Bits2/1, Extract Bits1/1
  Extract Bits16/1 -> Gain15/1
  Extract Bits14/1 -> Gain13/1
  Extract Bits15/1 -> Gain14/1
  Extract Bits13/1 -> Gain12/1
  Extract Bits12/1 -> Gain11/1
  Extract Bits11/1 -> Gain10/1
  Extract Bits9/1 -> Gain8/1
  Extract Bits10/1 -> Gain9/1
  Extract Bits2/1 -> Gain1/1
  Extract Bits5/1 -> Gain4/1
  Extract Bits1/1 -> Gain/1
  Extract Bits3/1 -> Gain2/1
  Extract Bits7/1 -> Gain6/1
  Extract Bits8/1 -> Gain7/1
  Extract Bits4/1 -> Gain3/1
  Extract Bits6/1 -> Gain5/1

== system CM13_2024a_MachE_for_UA_HIL/CarMaker_new/IPG Vehicle/Rototest and ORNL Interface/Get Wheel Spd Cmd Based on Wheel Dynamics/Whl Dynamics & Format CM Powertrain Signal/Diff Trq ==
  In1 : Inport
  Constant : Constant  Value=4.1
  Gain10 : Gain  Gain=0.5
  Product : Product  RndMeth=Zero
  Out1 : Outport
  wires:
  Gain10/1 -> Out1/1
  Constant/1 -> Product/1
  In1/1 -> Product/2
  Product/1 -> Gain10/1  "DiffTrq"

== system CM13_2024a_MachE_for_UA_HIL/CarMaker_new/IPG Vehicle/Rototest and ORNL Interface/Get Wheel Spd Cmd Based on Wheel Dynamics/Whl Dynamics & Format CM Powertrain Signal/Subsystem ==
  BrakeTorq : Inport
  <Car Trq_T2WFL> : Inport  Port=2
  AxlTorq : Inport  Port=3
  Constant : Constant  Value=0
  Discrete-Time Integrator : DiscreteIntegrator  IntegratorMethod=Integration: Backward Euler  InitialCondition=0/3.6/0.3235  SampleTime=0.001  ICPrevOutput=DiscIntNeverNeededParam  ICPrevScaledInput=DiscIntNeverNeededParam
  MATLAB Function : MATLAB Function  TreatAsAtomicUnit=on
  Memory : Memory
  Sum3 : Sum  Inputs=-++
  Switch : Switch  Criteria=u2 > Threshold  SaturateOnIntegerOverflow=off  InputSameDT=off
  WheelInertia : Subsystem
  rotv FL : Outport
  wires:
  Sum3/1 -> WheelInertia/1(In1)
  AxlTorq/1 -> MATLAB Function/1(axleTorq), Sum3/3
  <Car Trq_T2WFL>/1 -> Sum3/2
  BrakeTorq/1 -> Sum3/1
  Discrete-Time Integrator/1 -> Memory/1, rotv FL/1  "rotv FL"
  WheelInertia/1(Out1) -> Switch/3  "rota"
  MATLAB Function/1(switchFlag) -> Switch/2
  Switch/1 -> Discrete-Time Integrator/1
  Constant/1 -> Switch/1
  Memory/1 -> MATLAB Function/2(wheelSpd)

== system CM13_2024a_MachE_for_UA_HIL/CarMaker_new/IPG Vehicle/Rototest and ORNL Interface/Get Wheel Spd Cmd Based on Wheel Dynamics/Whl Dynamics & Format CM Powertrain Signal/Subsystem1 ==
  BrakeTorq : Inport
  <Car Trq_T2WFL> : Inport  Port=2
  AxlTorq : Inport  Port=3
  Discrete-Time Integrator : DiscreteIntegrator  IntegratorMethod=Integration: Backward Euler  InitialCondition=0/3.6/0.3235  SampleTime=0.001  ICPrevOutput=DiscIntNeverNeededParam  ICPrevScaledInput=DiscIntNeverNeededParam
  Sum3 : Sum  Inputs=-++
  WheelInertia : Subsystem
  rotv FL : Outport
  wires:
  Sum3/1 -> WheelInertia/1(In1)
  AxlTorq/1 -> Sum3/3
  <Car Trq_T2WFL>/1 -> Sum3/2
  BrakeTorq/1 -> Sum3/1
  Discrete-Time Integrator/1 -> rotv FL/1  "rotv FL"
  WheelInertia/1(Out1) -> Discrete-Time Integrator/1

== system CM13_2024a_MachE_for_UA_HIL/CarMaker_new/IPG Vehicle/Rototest and ORNL Interface/Get Wheel Spd Cmd Based on Wheel Dynamics/Whl Dynamics & Format CM Powertrain Signal/Subsystem2 ==
  BrakeTorq : Inport
  <Car Trq_T2WFR> : Inport  Port=2
  AxlTorq : Inport  Port=3
  Constant : Constant  Value=0
  Discrete-Time Integrator : DiscreteIntegrator  IntegratorMethod=Integration: Backward Euler  InitialCondition=0/3.6/0.3235  SampleTime=0.001  ICPrevOutput=DiscIntNeverNeededParam  ICPrevScaledInput=DiscIntNeverNeededParam
  MATLAB Function : MATLAB Function  TreatAsAtomicUnit=on
  Memory : Memory
  Sum3 : Sum  Inputs=-++
  Switch : Switch  Criteria=u2 > Threshold  SaturateOnIntegerOverflow=off  InputSameDT=off
  WheelInertia : Subsystem
  rotv FR : Outport
  wires:
  MATLAB Function/1(switchFlag) -> Switch/2
  Constant/1 -> Switch/1
  Switch/1 -> Discrete-Time Integrator/1
  WheelInertia/1(Out1) -> Switch/3  "rota"
  Discrete-Time Integrator/1 -> Memory/1, rotv FR/1  "rotv FL"
  AxlTorq/1 -> MATLAB Function/1(axleTorq), Sum3/3
  BrakeTorq/1 -> Sum3/1
  Sum3/1 -> WheelInertia/1(In1)
  <Car Trq_T2WFR>/1 -> Sum3/2
  Memory/1 -> MATLAB Function/2(wheelSpd)

== system CM13_2024a_MachE_for_UA_HIL/CarMaker_new/IPG Vehicle/Rototest and ORNL Interface/Get Wheel Spd Cmd Based on Wheel Dynamics/Whl Dynamics & Format CM Powertrain Signal/Subsystem3 ==
  BrakeTorq : Inport
  <Car Trq_T2WRL> : Inport  Port=2
  AxlTorq : Inport  Port=3
  Constant : Constant  Value=0
  Discrete-Time Integrator : DiscreteIntegrator  IntegratorMethod=Integration: Backward Euler  InitialCondition=0/3.6/0.3235  SampleTime=0.001  ICPrevOutput=DiscIntNeverNeededParam  ICPrevScaledInput=DiscIntNeverNeededParam
  MATLAB Function : MATLAB Function  TreatAsAtomicUnit=on
  Memory : Memory
  Sum3 : Sum  Inputs=-++
  Switch : Switch  Criteria=u2 > Threshold  SaturateOnIntegerOverflow=off  InputSameDT=off
  WheelInertia : Subsystem
  rotv RL : Outport
  wires:
  MATLAB Function/1(switchFlag) -> Switch/2
  Constant/1 -> Switch/1
  Switch/1 -> Discrete-Time Integrator/1
  WheelInertia/1(Out1) -> Switch/3  "rota"
  Discrete-Time Integrator/1 -> Memory/1, rotv RL/1  "rotv FL"
  AxlTorq/1 -> MATLAB Function/1(axleTorq), Sum3/3
  BrakeTorq/1 -> Sum3/1
  Sum3/1 -> WheelInertia/1(In1)
  <Car Trq_T2WRL>/1 -> Sum3/2
  Memory/1 -> MATLAB Function/2(wheelSpd)

== system CM13_2024a_MachE_for_UA_HIL/CarMaker_new/IPG Vehicle/Rototest and ORNL Interface/Get Wheel Spd Cmd Based on Wheel Dynamics/Whl Dynamics & Format CM Powertrain Signal/Subsystem4 ==
  BrakeTorq : Inport
  <Car Trq_T2WRR> : Inport  Port=2
  AxlTorq : Inport  Port=3
  Constant : Constant  Value=0
  Discrete-Time Integrator : DiscreteIntegrator  IntegratorMethod=Integration: Backward Euler  InitialCondition=0/3.6/0.3235  SampleTime=0.001  ICPrevOutput=DiscIntNeverNeededParam  ICPrevScaledInput=DiscIntNeverNeededParam
  MATLAB Function : MATLAB Function  TreatAsAtomicUnit=on
  Memory : Memory
  Sum3 : Sum  Inputs=-++
  Switch : Switch  Criteria=u2 > Threshold  SaturateOnIntegerOverflow=off  InputSameDT=off
  WheelInertia : Subsystem
  rotv RR : Outport
  wires:
  MATLAB Function/1(switchFlag) -> Switch/2
  Constant/1 -> Switch/1
  Switch/1 -> Discrete-Time Integrator/1
  WheelInertia/1(Out1) -> Switch/3  "rota"
  Discrete-Time Integrator/1 -> Memory/1, rotv RR/1  "rotv FL"
  AxlTorq/1 -> MATLAB Function/1(axleTorq), Sum3/3
  BrakeTorq/1 -> Sum3/1
  Sum3/1 -> WheelInertia/1(In1)
  <Car Trq_T2WRR>/1 -> Sum3/2
  Memory/1 -> MATLAB Function/2(wheelSpd)

== system CM13_2024a_MachE_for_UA_HIL/CarMaker_new/IPG Vehicle/Rototest and ORNL Interface/Get Wheel Spd Cmd Based on Wheel Dynamics/Whl Dynamics & Format CM Powertrain Signal/Subsystem5 ==
  In1 : Inport
  <Car Trq_T2WFR> : Inport  Port=2
  In3 : Inport  Port=3
  Discrete-Time Integrator1 : DiscreteIntegrator  IntegratorMethod=Integration: Backward Euler  InitialCondition=0/3.6/0.3235  SampleTime=0.001  ICPrevOutput=DiscIntNeverNeededParam  ICPrevScaledInput=DiscIntNeverNeededParam
  Sum2 : Sum  Inputs=-++
  WheelInertia1 : Subsystem
  rotv FR : Outport
  wires:
  <Car Trq_T2WFR>/1 -> Sum2/2
  Sum2/1 -> WheelInertia1/1(In1)
  In3/1 -> Sum2/3
  WheelInertia1/1(Out1) -> Discrete-Time Integrator1/1  "rota"
  In1/1 -> Sum2/1
  Discrete-Time Integrator1/1 -> rotv FR/1  "rotv FR"

== system CM13_2024a_MachE_for_UA_HIL/CarMaker_new/IPG Vehicle/Rototest and ORNL Interface/Get Wheel Spd Cmd Based on Wheel Dynamics/Whl Dynamics & Format CM Powertrain Signal/Subsystem6 ==
  In1 : Inport
  <Car Trq_T2WRL> : Inport  Port=2
  In3 : Inport  Port=3
  Discrete-Time Integrator2 : DiscreteIntegrator  IntegratorMethod=Integration: Backward Euler  InitialCondition=0/3.6/0.3235  SampleTime=0.001  ICPrevOutput=DiscIntNeverNeededParam  ICPrevScaledInput=DiscIntNeverNeededParam
  Sum : Sum  Inputs=-++
  WheelInertia2 : Subsystem
  rotv RL : Outport
  wires:
  In3/1 -> Sum/3
  WheelInertia2/1(Out1) -> Discrete-Time Integrator2/1  "rota"
  <Car Trq_T2WRL>/1 -> Sum/2
  Sum/1 -> WheelInertia2/1(In1)
  Discrete-Time Integrator2/1 -> rotv RL/1  "rotv RL"
  In1/1 -> Sum/1

== system CM13_2024a_MachE_for_UA_HIL/CarMaker_new/IPG Vehicle/Rototest and ORNL Interface/Get Wheel Spd Cmd Based on Wheel Dynamics/Whl Dynamics & Format CM Powertrain Signal/Subsystem7 ==
  In1 : Inport
  <Car Trq_T2WRR> : Inport  Port=2
  In3 : Inport  Port=3
  Discrete-Time Integrator3 : DiscreteIntegrator  IntegratorMethod=Integration: Backward Euler  InitialCondition=0/3.6/0.3235  SampleTime=0.001  ICPrevOutput=DiscIntNeverNeededParam  ICPrevScaledInput=DiscIntNeverNeededParam
  Sum1 : Sum  Inputs=-++
  WheelInertia3 : Subsystem
  rotv RR : Outport
  wires:
  Sum1/1 -> WheelInertia3/1(In1)
  WheelInertia3/1(Out1) -> Discrete-Time Integrator3/1  "rota"
  In3/1 -> Sum1/3
  <Car Trq_T2WRR>/1 -> Sum1/2
  In1/1 -> Sum1/1
  Discrete-Time Integrator3/1 -> rotv RR/1  "rotv RR"
